simulink model "kalman"  (R2021b)
settings: Solver=VariableStepAuto  StartTime=0.0  StopTime=10.0  RelTol=1e-3
values from neighbouring files (symbols this model uses):
  B_noise = [sysd.B ones(size(sysd.B,1),1)]    [Razzo27.m]
  C_states = eye(4)    [Razzo27.m]
  D_noise = [D_states zeros(size(D_states,1),1)]    [Razzo27.m]
  NK = zeros(4,3)    [Razzo27.m]
  RK = 10*blkdiag(1,1,1)    [Razzo27.m]
  sysd = c2d(sys,Ts)    [Razzo27.m]
  x0 = [deg2rad(0) deg2rad(-15) 0 200]    [Razzo27.m]
  x0K = [deg2rad(0) deg2rad(-20) 0 250]    [Razzo27.m]
  x2_max = deg2rad(20)    [Razzo27.m]
  x2_min = deg2rad(-20)    [Razzo27.m]
  x_ref = [0 0 0 0]'    [Razzo27.m]
undefined symbols (not defined in the file or in its folder): Discrete, mpc_point_5, N5, Q5, R5, S5, T_sampling, Time, u_max, u_min
libraries: simulink x2, ctrlSharedLib x1
settings Model: Creator=PaoloA  LastModifiedBy=PaoloA

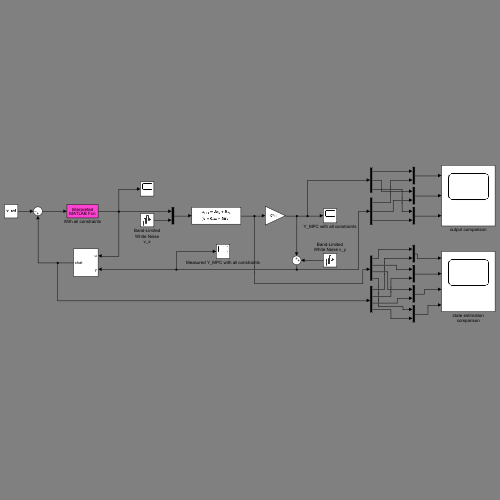
[thumbnail: Simulink's stored preview of the top-level diagram]
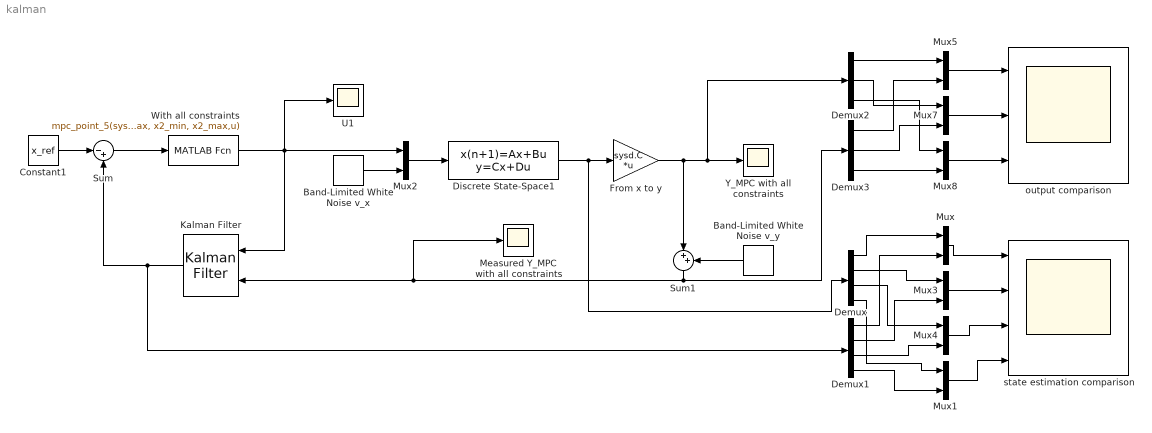
== system kalman ==
  "Band-Limited White Noise v_x " : simulink/Sources/Band-Limited White Noise  Cov=power_vx  Ts=T_sampling  seed=[23341]
  Band-Limited White Noise v_y : simulink/Sources/Band-Limited White Noise  Cov=power_vy  Ts=T_sampling  seed=[1258]
  Constant1 : Constant  Value=x_ref
  Demux : Demux
  Demux1 : Demux
  Demux2 : Demux  Outputs=3
  Demux3 : Demux  Outputs=3
  Discrete State-Space1 : DiscreteStateSpace  A=sysd.A  B=B_noise  C=C_states  D=D_noise  InitialCondition=x0  SampleTime=T_sampling
  From x to y : Gain  Gain=sysd.C  Multiplication=Matrix(K*u)
  Kalman Filter : ctrlSharedLib/Kalman Filter  TimeDomain=Discrete-Time  UseCurrentEstimator=off  ModelSource=Individual A, B, C, D matrices  ModelSourceVariable=ss(0.95,1,1,0,1)  A=sysd.A  B=sysd.B  C=sysd.C  D=sysd.D  NumberOfStates=1  NumberOfInputs=1  NumberOfOutputs=1  InitialEstimateSource=Dialog  X0=x0K  P0=10  UseK=off  UseGH=off  NumberOfProcessNoiseInputs=1  G=1  TimeInvariantG=on  H=0  TimeInvariantH=on  Q=QK  TimeInvariantQ=on  R=RK  TimeInvariantR=on  N=NK  TimeInvariantN=on  AddInputPort=on  AddEnablePort=off  OutputEstimatedY=off  OutputP=off  Ts=T_sampling
  Measured Y_MPC with all constraints : Scope
  Mux{,1..5,7..8} (8 alike) : Mux  Inputs=2
  Sum : Sum  Inputs=|-+
  Sum1 : Sum  Inputs=|++
  U1 : Scope
  With all constraints : MATLABFcn  MATLABFcn=mpc_point_5(sysd.A,sysd.B,Q5,R5,S5,N5,u_min,u_max, x2_min, x2_max,u)  OutputDimensions=1
  Y_MPC with all constraints : Scope
  output comparison : Scope  NumInputPorts=3
  "state estimation comparison " : Scope  NumInputPorts=4
  wires:
  "Band-Limited White Noise v_x "/1 -> Mux2/2
  Demux/4 -> Mux1/1
  Demux2/1 -> Mux5/1
  From x to y/1 -> Sum1/1, Demux2/1, Y_MPC with all constraints/1
  Demux2/2 -> Mux7/1
  Sum1/1 -> Measured Y_MPC with all constraints/1, Kalman Filter/2, Demux3/1
  Mux4/1 -> "state estimation comparison "/3
  Demux3/2 -> Mux7/2
  Demux3/1 -> Mux5/2
  Demux2/3 -> Mux8/1
  Demux1/2 -> Mux3/2
  Demux3/3 -> Mux8/2
  Mux5/1 -> output comparison/1
  Constant1/1 -> Sum/1
  Demux1/4 -> Mux1/2
  Band-Limited White Noise v_y/1 -> Sum1/2
  Mux2/1 -> Discrete State-Space1/1
  Mux8/1 -> output comparison/3
  With all constraints/1 -> Kalman Filter/1, Mux2/1, U1/1
  Mux/1 -> "state estimation comparison "/1
  Mux7/1 -> output comparison/2
  Demux/1 -> Mux/1
  Kalman Filter/1 -> Demux1/1, Sum/2
  Mux1/1 -> "state estimation comparison "/4
  Demux1/1 -> Mux/2
  Discrete State-Space1/1 -> From x to y/1, Demux/1
  Demux/3 -> Mux4/1
  Demux/2 -> Mux3/1
  Sum/1 -> With all constraints/1
  Demux1/3 -> Mux4/2
  Mux3/1 -> "state estimation comparison "/2
